simulink model "a1be3de"  (R2022a)
settings: Solver=VariableStepAuto  StartTime=0.0  StopTime=10.0  RelTol=1e-3
model workspace (MAT data in the model file):
  M_B = 5500
  lambda_max = 0.13
values from neighbouring files (symbols this model uses):
  b = 0.36    [a1be3ab.mat]
  c1 = 0.86    [a1be3ab.mat]
  c2 = 33.82    [a1be3ab.mat]
  c3 = 0.36    [a1be3ab.mat]
  g = 9.81    [a1be3ab.mat]
  J_R = 0.8    [a1be3ab.mat]
  m = 1500    [a1be3ab.mat]
  r_R = 0.3    [a1be3ab.mat]
settings Model: Creator=attit  LastModifiedBy=attit

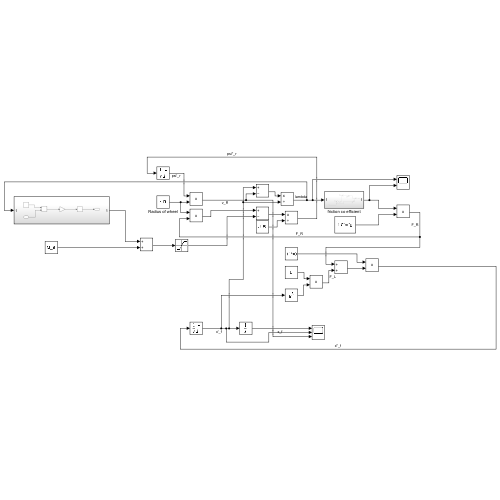
[thumbnail: Simulink's stored preview of the top-level diagram]
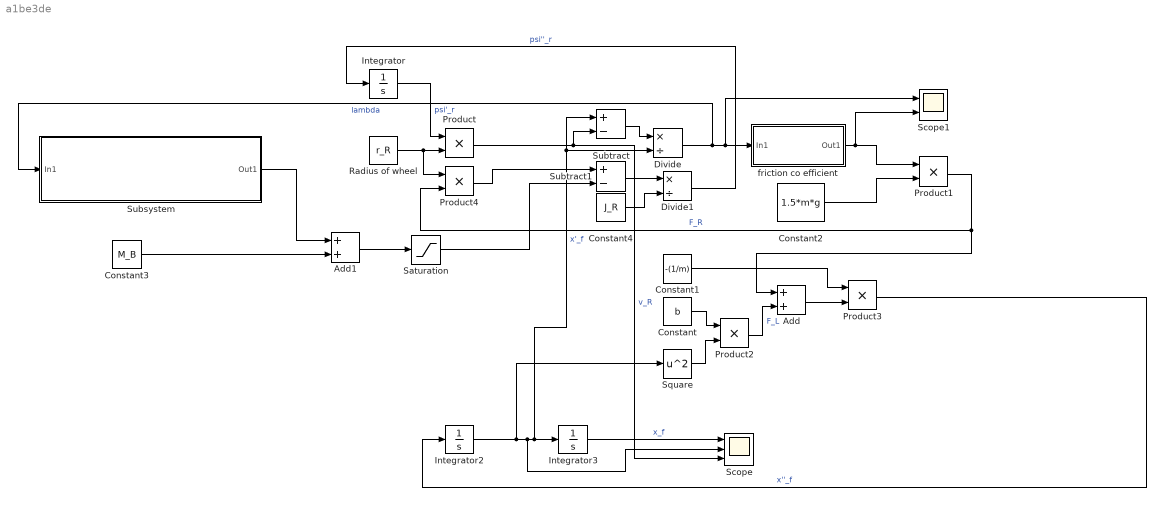
== system a1be3de ==
  Add : Sum
  Add1 : Sum
  Constant : Constant  Value=b
  Constant1 : Constant  Value=-(1/m)
  Constant2 : Constant  Value=1.5*m*g
  Constant3 : Constant  Value=M_B
  Constant4 : Constant  Value=J_R
  Divide : Product  Inputs=*/
  Divide1 : Product  Inputs=*/
  Integrator : Integrator  InitialCondition=100  LimitOutput=on  LowerSaturationLimit=0
  Integrator2 : Integrator  InitialCondition=30  LimitOutput=on  LowerSaturationLimit=0
  Integrator3 : Integrator
  Product{,1..4} (5 alike) : Product
  Radius of wheel : Constant  Value=r_R
  Saturation : Saturate  UpperLimit=10000  LowerLimit=0
  Scope : Scope  NumInputPorts=3
  Scope1 : Scope  NumInputPorts=2
  Square : Math  Operator=square
  Subsystem : Subsystem
  Subtract : Sum  Inputs=+-
  Subtract1 : Sum  Inputs=+-
  friction co efficient : Subsystem
  wires:
  Constant4/1 -> Divide1/2
  Product/1 -> Scope/3, Subtract/2  "v_R"
  Product3/1 -> Integrator2/1  "x''_f"
  Constant/1 -> Product2/1
  Subtract1/1 -> Divide1/1
  Add/1 -> Product3/2
  friction co efficient/1(Out1) -> Scope1/2, Product1/1
  Square/1 -> Product2/2
  Integrator3/1 -> Scope/1  "x_f"
  Product2/1 -> Add/2  "F_L"
  Product1/1 -> Add/1, Product4/2  "F_R"
  Divide/1 -> Subsystem/1(In1), Scope1/1, friction co efficient/1(In1)  "lambda"
  Constant2/1 -> Product1/2
  Subtract/1 -> Divide/1
  Integrator2/1 -> Square/1, Scope/2, Divide/2, Subtract/1, Integrator3/1  "x'_f"
  Radius of wheel/1 -> Product4/1, Product/2
  Divide1/1 -> Integrator/1  "psi''_r"
  Constant1/1 -> Product3/1
  Integrator/1 -> Product/1  "psi'_r"
  Product4/1 -> Subtract1/1
  Subsystem/1(Out1) -> Add1/1
  Constant3/1 -> Add1/2
  Add1/1 -> Saturation/1
  Saturation/1 -> Subtract1/2

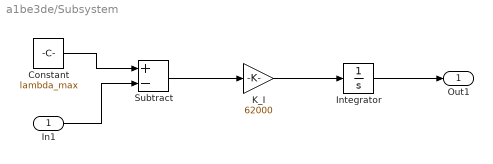
== system a1be3de/Subsystem ==
  In1 : Inport
  Constant : Constant  Value=lambda_max
  Integrator : Integrator
  K_I : Gain  Gain=62000
  Subtract : Sum  Inputs=+-
  Out1 : Outport
  wires:
  Constant/1 -> Subtract/1
  In1/1 -> Subtract/2
  Subtract/1 -> K_I/1
  K_I/1 -> Integrator/1
  Integrator/1 -> Out1/1

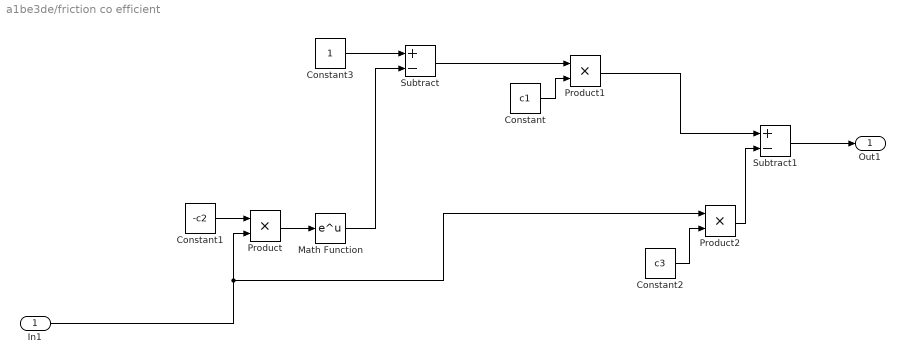
== system a1be3de/friction co efficient ==
  In1 : Inport
  Constant : Constant  Value=c1
  Constant1 : Constant  Value=-c2
  Constant2 : Constant  Value=c3
  Constant3 : Constant
  Math Function : Math  SignedPower=on  RndMeth=Zero
  Product : Product
  Product1 : Product
  Product2 : Product
  Subtract : Sum  Inputs=+-
  Subtract1 : Sum  Inputs=+-
  Out1 : Outport
  wires:
  Constant1/1 -> Product/1
  In1/1 -> Product/2, Product2/1
  Product/1 -> Math Function/1
  Math Function/1 -> Subtract/2
  Constant3/1 -> Subtract/1
  Subtract/1 -> Product1/1
  Constant/1 -> Product1/2
  Constant2/1 -> Product2/2
  Product1/1 -> Subtract1/1
  Product2/1 -> Subtract1/2
  Subtract1/1 -> Out1/1
